simulink model "sim_complete_statespace"  (R2023b)
settings: Solver=VariableStepAuto  StartTime=0.0  StopTime=100.0  RelTol=1e-3
settings Model: Creator=Jhchen  LastModifiedBy=Jhchen

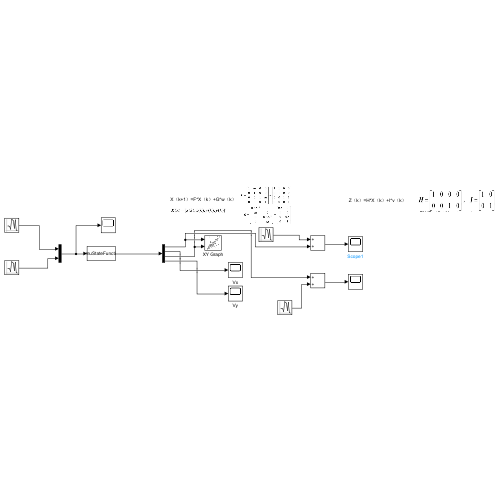
[thumbnail: Simulink's stored preview of the top-level diagram]
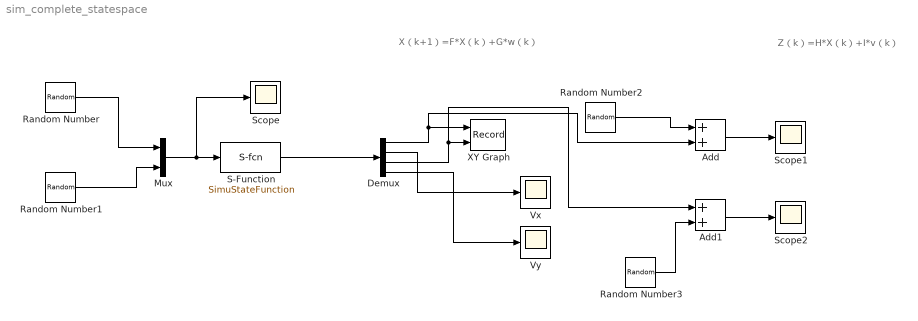
== system sim_complete_statespace ==
  note: Z（k）=H*X（k）+I*v（k）
  note: X（k+1）=F*X（k）+G*w（k）
  Add : Sum
  Add1 : Sum
  Demux : Demux
  Mux : Mux  Inputs=2
  Random Number : RandomNumber  Variance=0.01  SampleTime=1
  Random Number1 : RandomNumber  Variance=0.09  SampleTime=1
  Random Number2 : RandomNumber  Variance=0.04  SampleTime=1
  Random Number3 : RandomNumber  Variance=0.04  SampleTime=1
  S-Function : S-Function  FunctionName=SimuStateFunction  SFunctionDeploymentMode=off  EnableBusSupport=off
  Scope : Scope
  Scope1 : Scope
  Scope2 : Scope
  Vx : Scope
  Vy : Scope
  XY Graph : Record  FileSettingsInternal="{\"entries\":[{\"content\":{\"excelSettings\":{\"content\":{},\"type\":\"Streamout.ExcelSettings\"}},\"type\":\"Streamout.FileSettingStorage\",\"uuid\":\"\"}],\"packageUris\":[\"http:\\/\\/schema.mathworks.com\\/mf0\\/streamout_blocks\\/R2020a\"],\"version\":\"1.0\"}"  Layout=[1 1]  SignalsInternal="{\"entries\":[{\"content\":{\"signals\":[{\"content\":{\"blockPath\":[],\"dimensions\":[1],\"domain\":\"\",\"lineColor\":\"#a2142f\",\"plots\":[1],\"port\":1,\"sid\":[\"\"],\"signalID\":166,\"signalName\":\"Demux:1\"},\"type\":\"RecordBlkView.Signal\",\"uuid\":\"\"},{\"content\":{\"blockPath\":[],\"dimensions\":[1],\"domain\":\"\",\"lineColor\":\"#139fff\",\"plots\":[1],\"port\":2,\"sid\":[\"\"],\"signalID\":170,\"signalName\":\"Demux:3\"},\"type\":\"RecordBlkView.Signal\",\"uuid\":\"\"}]},\"type\":\"RecordBlkView.InputSignals\",\"uuid\":\"\"}],\"packageUris\":[\"http:\\/\\/schema.mathworks.com\\/mf0\\/streamout_blocks\\/R2020a\"],\"version\":\"1.0\"}"  VisualizationBindings="{\"xyplotplugin\":{\"info\":[{\"series\":[{\"bindingParametersList\":[{\"parameter\":\"X-Axis\",\"signalID\":166,\"signalName\":\"Demux:1\"},{\"parameter\":\"Y-Axis\",\"signalID\":170,\"signalName\":\"Demux:3\"}],\"seriesID\":38470}],\"subplotID\":1}]}}"  CompatibilityTag=XY
  wires:
  Random Number1/1 -> Mux/2
  Random Number/1 -> Mux/1
  Mux/1 -> Scope/1, S-Function/1
  S-Function/1 -> Demux/1
  Demux/1 -> Add/2, XY Graph/1
  Demux/3 -> Add1/1, XY Graph/2
  Demux/4 -> Vy/1
  Demux/2 -> Vx/1
  Random Number2/1 -> Add/1
  Random Number3/1 -> Add1/2
  Add1/1 -> Scope2/1
  Add/1 -> Scope1/1
